simulink model "PRBS_Para_BackgroundSim"  (R2015a)
settings: Solver=ode5  StartTime=0.0  StopTime=10  FixedStep=sim_stepSize
undefined symbols (not defined in the file or in its folder): sim_external, sim_Qgain, sim_releaseRate, sim_zoneVolGain
settings Model: Creator=David  LastModifiedBy=davidveitch
settings SolverCC: NumberNewtonIterations=4  MaxConsecutiveMinStep=auto
settings DataIOCC: LimitDataPoints=off  SaveOutput=off  SignalLogging=off  DSMLogging=off  SaveTime=off  TimeSaveName=d_toutPRBS  OutputSaveName=Conc
settings OptimizationCC: ExpressionDepthLimit=2147483647  SimCompilerOptimization=on
settings DebuggingCC: UnderspecifiedInitializationDetection=Classic  MergeDetectMultiDrivingBlocksExec=none  SolverPrmCheckMsg=warning  FcnCallInpInsideContextMsg=EnableAllAsWarning  StateNameClashWarn=warning
settings ModelReferenceCC: UpdateModelReferenceTargets=IfOutOfDate
settings SFSimCC: SFSimEcho=off

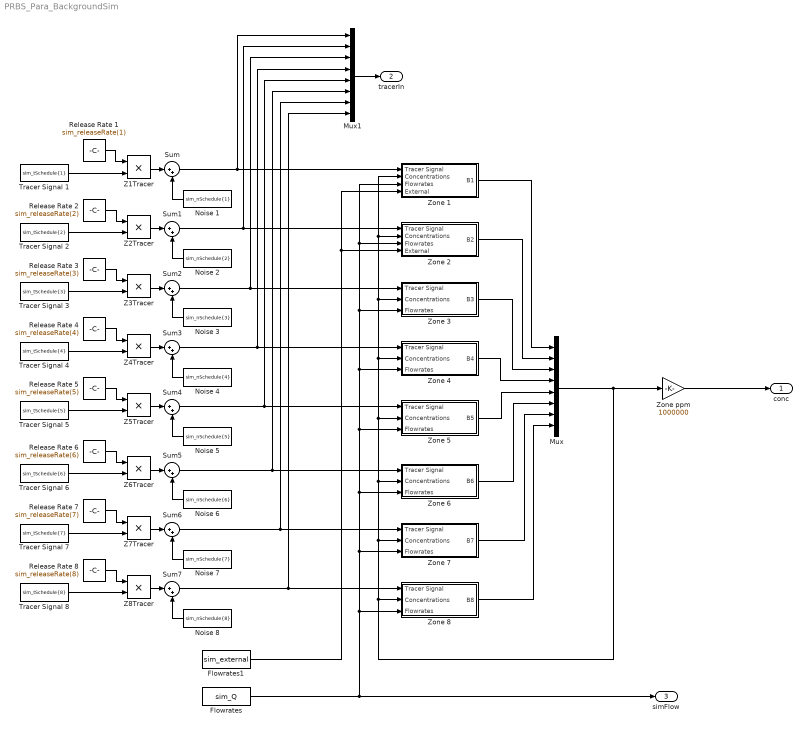
== system PRBS_Para_BackgroundSim ==
  Flowrates : FromWorkspace  VariableName=sim_Q  SampleTime=0  OutputAfterFinalValue=Holding final value
  Flowrates1 : FromWorkspace  VariableName=sim_external  SampleTime=0  OutputAfterFinalValue=Holding final value
  Mux : Mux  Inputs=8
  Mux1 : Mux  Inputs=8
  Noise 1 : FromWorkspace  VariableName=sim_nSchedule{1}  SampleTime=0  Interpolate=off  OutputAfterFinalValue=Holding final value
  Noise 2 : FromWorkspace  VariableName=sim_nSchedule{2}  SampleTime=0  Interpolate=off  OutputAfterFinalValue=Holding final value
  Noise 3 : FromWorkspace  VariableName=sim_nSchedule{3}  SampleTime=0  Interpolate=off  OutputAfterFinalValue=Holding final value
  "Noise 4 " : FromWorkspace  VariableName=sim_nSchedule{4}  SampleTime=0  Interpolate=off  OutputAfterFinalValue=Holding final value
  Noise 5 : FromWorkspace  VariableName=sim_nSchedule{5}  SampleTime=0  Interpolate=off  OutputAfterFinalValue=Holding final value
  Noise 6 : FromWorkspace  VariableName=sim_nSchedule{6}  SampleTime=0  Interpolate=off  OutputAfterFinalValue=Holding final value
  Noise 7 : FromWorkspace  VariableName=sim_nSchedule{7}  SampleTime=0  Interpolate=off  OutputAfterFinalValue=Holding final value
  Noise 8 : FromWorkspace  VariableName=sim_nSchedule{8}  SampleTime=0  Interpolate=off  OutputAfterFinalValue=Holding final value
  Release Rate 1 : Constant  Value=sim_releaseRate(1)
  Release Rate 2 : Constant  Value=sim_releaseRate(2)
  Release Rate 3 : Constant  Value=sim_releaseRate(3)
  Release Rate 4 : Constant  Value=sim_releaseRate(4)
  Release Rate 5 : Constant  Value=sim_releaseRate(5)
  Release Rate 6 : Constant  Value=sim_releaseRate(6)
  Release Rate 7 : Constant  Value=sim_releaseRate(7)
  Release Rate 8 : Constant  Value=sim_releaseRate(8)
  Sum{,1..7} (8 alike) : Sum  Inputs=|++
  Tracer Signal 1 : FromWorkspace  VariableName=sim_tSchedule{1}  SampleTime=0  Interpolate=off  OutputAfterFinalValue=Holding final value
  Tracer Signal 2 : FromWorkspace  VariableName=sim_tSchedule{2}  SampleTime=0  Interpolate=off  OutputAfterFinalValue=Holding final value
  Tracer Signal 3 : FromWorkspace  VariableName=sim_tSchedule{3}  SampleTime=0  Interpolate=off  OutputAfterFinalValue=Holding final value
  Tracer Signal 4 : FromWorkspace  VariableName=sim_tSchedule{4}  SampleTime=0  Interpolate=off  OutputAfterFinalValue=Holding final value
  Tracer Signal 5 : FromWorkspace  VariableName=sim_tSchedule{5}  SampleTime=0  Interpolate=off  OutputAfterFinalValue=Holding final value
  Tracer Signal 6 : FromWorkspace  VariableName=sim_tSchedule{6}  SampleTime=0  Interpolate=off  OutputAfterFinalValue=Holding final value
  Tracer Signal 7 : FromWorkspace  VariableName=sim_tSchedule{7}  SampleTime=0  Interpolate=off  OutputAfterFinalValue=Holding final value
  Tracer Signal 8 : FromWorkspace  VariableName=sim_tSchedule{8}  SampleTime=0  Interpolate=off  OutputAfterFinalValue=Holding final value
  Z1Tracer : Product  RndMeth=Zero
  Z2Tracer : Product  RndMeth=Zero
  Z3Tracer : Product  RndMeth=Zero
  Z4Tracer : Product  RndMeth=Zero
  Z5Tracer : Product  RndMeth=Zero
  Z6Tracer : Product  RndMeth=Zero
  Z7Tracer : Product  RndMeth=Zero
  Z8Tracer : Product  RndMeth=Zero
  Zone ppm : Gain  Gain=1000000
  Zone 1 : Subsystem
  Zone 2 : Subsystem
  Zone 3 : Subsystem
  Zone 4 : Subsystem
  Zone 5 : Subsystem
  Zone 6 : Subsystem
  Zone 7 : Subsystem
  Zone 8 : Subsystem
  conc : Outport
  tracerIn : Outport  Port=2
  simFlow : Outport  Port=3
  wires:
  Zone 1/1(B1) -> Mux/1
  Zone 2/1(B2) -> Mux/2
  Zone 3/1(B3) -> Mux/3
  Zone ppm/1 -> conc/1
  Release Rate 1/1 -> Z1Tracer/1
  Tracer Signal 1/1 -> Z1Tracer/2
  Tracer Signal 2/1 -> Z2Tracer/2
  Tracer Signal 3/1 -> Z3Tracer/2
  Flowrates/1 -> simFlow/1, Zone 8/3(Flowrates), Zone 7/3(Flowrates), Zone 6/3(Flowrates), Zone 1/3(Flowrates), Zone 2/3(Flowrates), Zone 3/3(Flowrates), Zone 4/3(Flowrates), Zone 5/3(Flowrates)
  Noise 1/1 -> Sum/2
  Sum/1 -> Mux1/1, Zone 1/1(Tracer Signal)
  Z1Tracer/1 -> Sum/1
  Sum1/1 -> Mux1/2, Zone 2/1(Tracer Signal)
  Sum2/1 -> Mux1/3, Zone 3/1(Tracer Signal)
  Noise 2/1 -> Sum1/2
  Noise 3/1 -> Sum2/2
  Z3Tracer/1 -> Sum2/1
  Z2Tracer/1 -> Sum1/1
  Tracer Signal 4/1 -> Z4Tracer/2
  Sum3/1 -> Mux1/4, Zone 4/1(Tracer Signal)
  "Noise 4 "/1 -> Sum3/2
  Z4Tracer/1 -> Sum3/1
  Tracer Signal 5/1 -> Z5Tracer/2
  Sum4/1 -> Mux1/5, Zone 5/1(Tracer Signal)
  Noise 5/1 -> Sum4/2
  Z5Tracer/1 -> Sum4/1
  Zone 4/1(B4) -> Mux/4
  Zone 5/1(B5) -> Mux/5
  Mux1/1 -> tracerIn/1
  Tracer Signal 6/1 -> Z6Tracer/2
  Sum5/1 -> Mux1/6, Zone 6/1(Tracer Signal)
  Noise 6/1 -> Sum5/2
  Z6Tracer/1 -> Sum5/1
  Tracer Signal 7/1 -> Z7Tracer/2
  Sum6/1 -> Mux1/7, Zone 7/1(Tracer Signal)
  Noise 7/1 -> Sum6/2
  Z7Tracer/1 -> Sum6/1
  Tracer Signal 8/1 -> Z8Tracer/2
  Sum7/1 -> Mux1/8, Zone 8/1(Tracer Signal)
  Noise 8/1 -> Sum7/2
  Z8Tracer/1 -> Sum7/1
  Zone 6/1(B6) -> Mux/6
  Zone 7/1(B7) -> Mux/7
  Zone 8/1(B8) -> Mux/8
  Release Rate 3/1 -> Z3Tracer/1
  Release Rate 4/1 -> Z4Tracer/1
  Release Rate 5/1 -> Z5Tracer/1
  Release Rate 6/1 -> Z6Tracer/1
  Release Rate 7/1 -> Z7Tracer/1
  Release Rate 8/1 -> Z8Tracer/1
  Release Rate 2/1 -> Z2Tracer/1
  Flowrates1/1 -> Zone 2/4(External), Zone 1/4(External)
  Mux/1 -> Zone ppm/1, Zone 8/2(Concentrations), Zone 7/2(Concentrations), Zone 6/2(Concentrations), Zone 5/2(Concentrations), Zone 4/2(Concentrations), Zone 3/2(Concentrations), Zone 2/2(Concentrations), Zone 1/2(Concentrations)

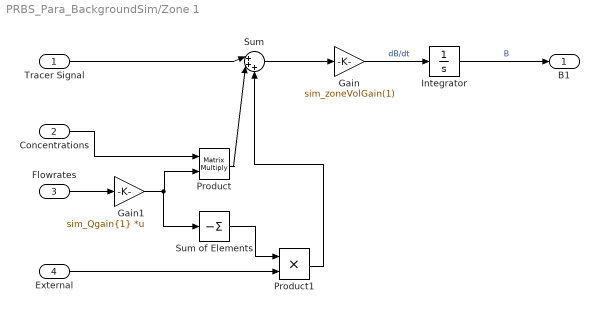
== system PRBS_Para_BackgroundSim/Zone 1 ==
  Tracer Signal : Inport
  Concentrations : Inport  Port=2
  Flowrates : Inport  Port=3
  External : Inport  Port=4
  Gain : Gain  Gain=sim_zoneVolGain(1)
  Gain1 : Gain  Gain=sim_Qgain{1}  Multiplication=Matrix(K*u)
  Integrator : Integrator  InitialCondition=sim_external(1,2)
  Product : Product  Multiplication=Matrix(*)  RndMeth=Zero
  Product1 : Product  RndMeth=Zero
  Sum : Sum  Inputs=|+++
  Sum of Elements : Sum  Inputs=-
  B1 : Outport
  wires:
  Sum/1 -> Gain/1
  Gain/1 -> Integrator/1  "dB/dt"
  Integrator/1 -> B1/1  "B"
  Concentrations/1 -> Product/1
  Product/1 -> Sum/2
  Tracer Signal/1 -> Sum/1
  Flowrates/1 -> Gain1/1
  Gain1/1 -> Sum of Elements/1, Product/2
  External/1 -> Product1/2
  Sum of Elements/1 -> Product1/1
  Product1/1 -> Sum/3

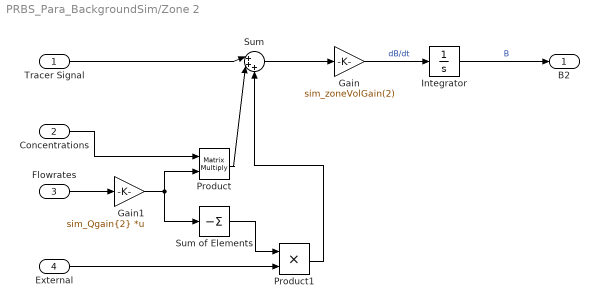
== system PRBS_Para_BackgroundSim/Zone 2 ==
  Tracer Signal : Inport
  Concentrations : Inport  Port=2
  Flowrates : Inport  Port=3
  External : Inport  Port=4
  Gain : Gain  Gain=sim_zoneVolGain(2)
  Gain1 : Gain  Gain=sim_Qgain{2}  Multiplication=Matrix(K*u)
  Integrator : Integrator  InitialCondition=sim_external(1,2)
  Product : Product  Multiplication=Matrix(*)  RndMeth=Zero
  Product1 : Product  RndMeth=Zero
  Sum : Sum  Inputs=|+++
  Sum of Elements : Sum  Inputs=-
  B2 : Outport
  wires:
  Sum/1 -> Gain/1
  Gain/1 -> Integrator/1  "dB/dt"
  Integrator/1 -> B2/1  "B"
  Concentrations/1 -> Product/1
  Product/1 -> Sum/2
  Tracer Signal/1 -> Sum/1
  Flowrates/1 -> Gain1/1
  Gain1/1 -> Sum of Elements/1, Product/2
  External/1 -> Product1/2
  Sum of Elements/1 -> Product1/1
  Product1/1 -> Sum/3

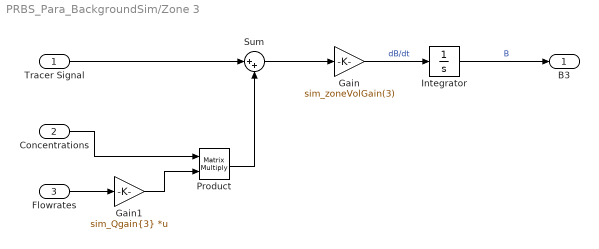
== system PRBS_Para_BackgroundSim/Zone 3 ==
  Tracer Signal : Inport
  Concentrations : Inport  Port=2
  Flowrates : Inport  Port=3
  Gain : Gain  Gain=sim_zoneVolGain(3)
  Gain1 : Gain  Gain=sim_Qgain{3}  Multiplication=Matrix(K*u)
  Integrator : Integrator
  Product : Product  Multiplication=Matrix(*)  RndMeth=Zero
  Sum : Sum  Inputs=|++
  B3 : Outport
  wires:
  Sum/1 -> Gain/1
  Gain/1 -> Integrator/1  "dB/dt"
  Integrator/1 -> B3/1  "B"
  Concentrations/1 -> Product/1
  Product/1 -> Sum/2
  Tracer Signal/1 -> Sum/1
  Flowrates/1 -> Gain1/1
  Gain1/1 -> Product/2

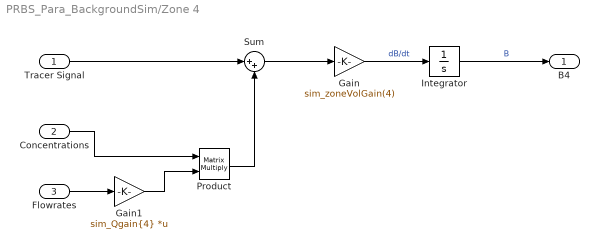
== system PRBS_Para_BackgroundSim/Zone 4 ==
  Tracer Signal : Inport
  Concentrations : Inport  Port=2
  Flowrates : Inport  Port=3
  Gain : Gain  Gain=sim_zoneVolGain(4)
  Gain1 : Gain  Gain=sim_Qgain{4}  Multiplication=Matrix(K*u)
  Integrator : Integrator
  Product : Product  Multiplication=Matrix(*)  RndMeth=Zero
  Sum : Sum  Inputs=|++
  B4 : Outport
  wires:
  Sum/1 -> Gain/1
  Gain/1 -> Integrator/1  "dB/dt"
  Integrator/1 -> B4/1  "B"
  Concentrations/1 -> Product/1
  Product/1 -> Sum/2
  Tracer Signal/1 -> Sum/1
  Flowrates/1 -> Gain1/1
  Gain1/1 -> Product/2

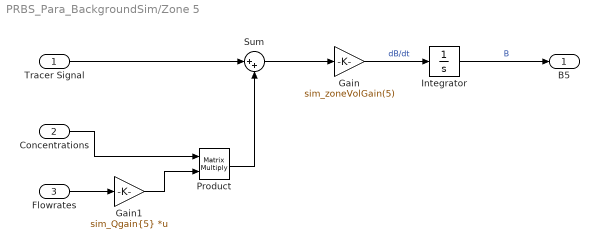
== system PRBS_Para_BackgroundSim/Zone 5 ==
  Tracer Signal : Inport
  Concentrations : Inport  Port=2
  Flowrates : Inport  Port=3
  Gain : Gain  Gain=sim_zoneVolGain(5)
  Gain1 : Gain  Gain=sim_Qgain{5}  Multiplication=Matrix(K*u)
  Integrator : Integrator
  Product : Product  Multiplication=Matrix(*)  RndMeth=Zero
  Sum : Sum  Inputs=|++
  B5 : Outport
  wires:
  Sum/1 -> Gain/1
  Gain/1 -> Integrator/1  "dB/dt"
  Integrator/1 -> B5/1  "B"
  Concentrations/1 -> Product/1
  Product/1 -> Sum/2
  Tracer Signal/1 -> Sum/1
  Flowrates/1 -> Gain1/1
  Gain1/1 -> Product/2

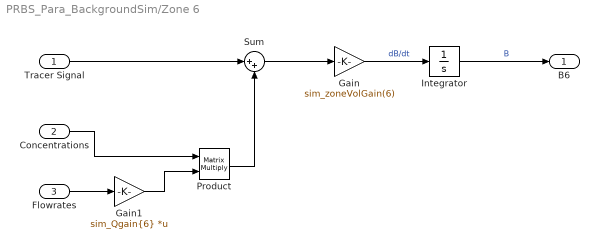
== system PRBS_Para_BackgroundSim/Zone 6 ==
  Tracer Signal : Inport
  Concentrations : Inport  Port=2
  Flowrates : Inport  Port=3
  Gain : Gain  Gain=sim_zoneVolGain(6)
  Gain1 : Gain  Gain=sim_Qgain{6}  Multiplication=Matrix(K*u)
  Integrator : Integrator
  Product : Product  Multiplication=Matrix(*)  RndMeth=Zero
  Sum : Sum  Inputs=|++
  B6 : Outport
  wires:
  Sum/1 -> Gain/1
  Gain/1 -> Integrator/1  "dB/dt"
  Integrator/1 -> B6/1  "B"
  Concentrations/1 -> Product/1
  Product/1 -> Sum/2
  Tracer Signal/1 -> Sum/1
  Flowrates/1 -> Gain1/1
  Gain1/1 -> Product/2

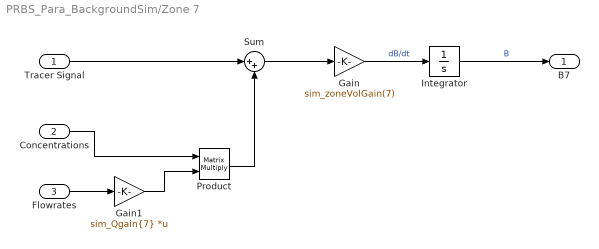
== system PRBS_Para_BackgroundSim/Zone 7 ==
  Tracer Signal : Inport
  Concentrations : Inport  Port=2
  Flowrates : Inport  Port=3
  Gain : Gain  Gain=sim_zoneVolGain(7)
  Gain1 : Gain  Gain=sim_Qgain{7}  Multiplication=Matrix(K*u)
  Integrator : Integrator
  Product : Product  Multiplication=Matrix(*)  RndMeth=Zero
  Sum : Sum  Inputs=|++
  B7 : Outport
  wires:
  Sum/1 -> Gain/1
  Gain/1 -> Integrator/1  "dB/dt"
  Integrator/1 -> B7/1  "B"
  Concentrations/1 -> Product/1
  Product/1 -> Sum/2
  Tracer Signal/1 -> Sum/1
  Flowrates/1 -> Gain1/1
  Gain1/1 -> Product/2

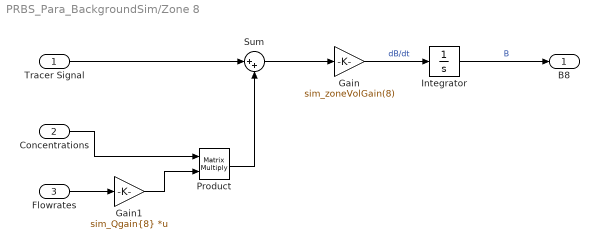
== system PRBS_Para_BackgroundSim/Zone 8 ==
  Tracer Signal : Inport
  Concentrations : Inport  Port=2
  Flowrates : Inport  Port=3
  Gain : Gain  Gain=sim_zoneVolGain(8)
  Gain1 : Gain  Gain=sim_Qgain{8}  Multiplication=Matrix(K*u)
  Integrator : Integrator
  Product : Product  Multiplication=Matrix(*)  RndMeth=Zero
  Sum : Sum  Inputs=|++
  B8 : Outport
  wires:
  Sum/1 -> Gain/1
  Gain/1 -> Integrator/1  "dB/dt"
  Integrator/1 -> B8/1  "B"
  Concentrations/1 -> Product/1
  Product/1 -> Sum/2
  Tracer Signal/1 -> Sum/1
  Flowrates/1 -> Gain1/1
  Gain1/1 -> Product/2
